simulink model "Differential_InWheel_RW_Torque_vectoring_control"  (R2020a)
settings: Solver=VariableStepAuto  StartTime=0.0  StopTime=Ts  RelTol=1e-3
values from neighbouring files (symbols this model uses):
  B1 = 1.200    (= 1.2)    [TVC_Parameters.m]
  ki = 0.2    [TVC_Parameters.m]
  kp = 1    [TVC_Parameters.m]
  m = 235    [TVC_Parameters.m]
  R = 0.3    [TVC_Parameters.m]
  Tin = 21    [TVC_Parameters.m]
  Ts = 1e-06    [TVC_Parameters.m]
libraries: simulink_extras x3, autolibshared x3, vehdynlibsteering x1, autolibshareddiff x1, autolibsharedcoupling x1
(part 2 of 2)

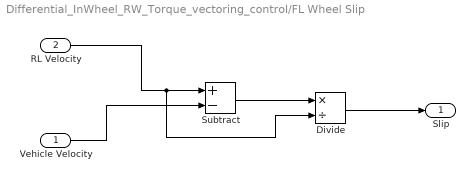
== system Differential_InWheel_RW_Torque_vectoring_control/FL Wheel Slip ==
  Vehicle Velocity : Inport
  RL Velocity : Inport  Port=2
  Divide : Product  Inputs=*/
  Subtract : Sum  Inputs=+-
  "Slip " : Outport
  wires:
  Divide/1 -> "Slip "/1
  Subtract/1 -> Divide/1
  Vehicle Velocity/1 -> Subtract/2
  RL Velocity/1 -> Subtract/1, Divide/2

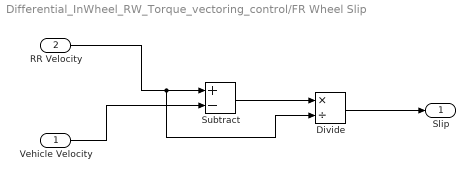
== system Differential_InWheel_RW_Torque_vectoring_control/FR Wheel Slip ==
  Vehicle Velocity : Inport
  RR Velocity : Inport  Port=2
  Divide : Product  Inputs=*/
  Subtract : Sum  Inputs=+-
  Slip : Outport
  wires:
  RR Velocity/1 -> Divide/2, Subtract/1
  Vehicle Velocity/1 -> Subtract/2
  Subtract/1 -> Divide/1
  Divide/1 -> Slip/1

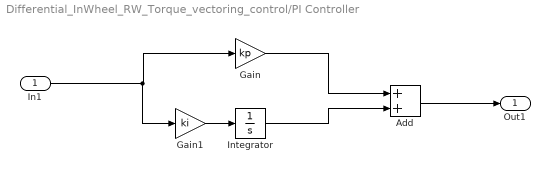
== system Differential_InWheel_RW_Torque_vectoring_control/PI Controller ==
  In1 : Inport
  Add : Sum
  Gain : Gain  Gain=kp
  Gain1 : Gain  Gain=ki
  Integrator : Integrator
  Out1 : Outport
  wires:
  Gain/1 -> Add/1
  Integrator/1 -> Add/2
  In1/1 -> Gain1/1, Gain/1
  Add/1 -> Out1/1
  Gain1/1 -> Integrator/1

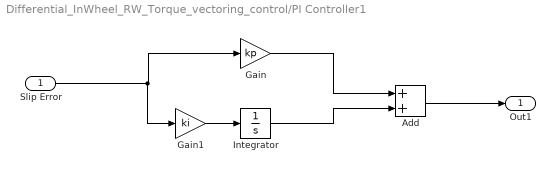
== system Differential_InWheel_RW_Torque_vectoring_control/PI Controller1 ==
  Slip Error : Inport
  Add : Sum
  Gain : Gain  Gain=kp
  Gain1 : Gain  Gain=ki
  Integrator : Integrator
  Out1 : Outport
  wires:
  Add/1 -> Out1/1
  Slip Error/1 -> Gain/1, Gain1/1
  Integrator/1 -> Add/2
  Gain/1 -> Add/1
  Gain1/1 -> Integrator/1

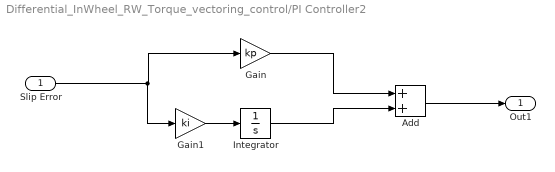
== system Differential_InWheel_RW_Torque_vectoring_control/PI Controller2 ==
  Slip Error : Inport
  Add : Sum
  Gain : Gain  Gain=kp
  Gain1 : Gain  Gain=ki
  Integrator : Integrator
  Out1 : Outport
  wires:
  Gain/1 -> Add/1
  Integrator/1 -> Add/2
  Slip Error/1 -> Gain1/1, Gain/1
  Add/1 -> Out1/1
  Gain1/1 -> Integrator/1

== matlab function Differential_InWheel_RW_Torque_vectoring_control/MATLAB Function ==
  data: u input; y output; v input; w input
function y = fcn(u,v,w)
v_r=sqrt(u^2+v^2+w^2);
y = v_r;

== matlab function Differential_InWheel_RW_Torque_vectoring_control/MATLAB Function1 ==
  data: u input; y output; v input
function y = fcn(u,v)
L=4;
Rt=L*cot((u+v)/2);

y = Rt;
